simulink subsystem "rotorTemp"  (R2022b)
settings: Solver=VariableStepAuto  StartTime=0.0  StopTime=10.0  RelTol=1e-3
libraries: rotors x4
settings Model: Creator=serga  LastModifiedBy=serga

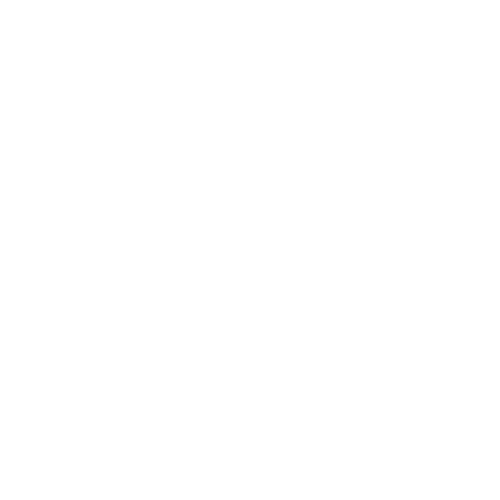
[thumbnail: Simulink's stored preview of the top-level diagram]
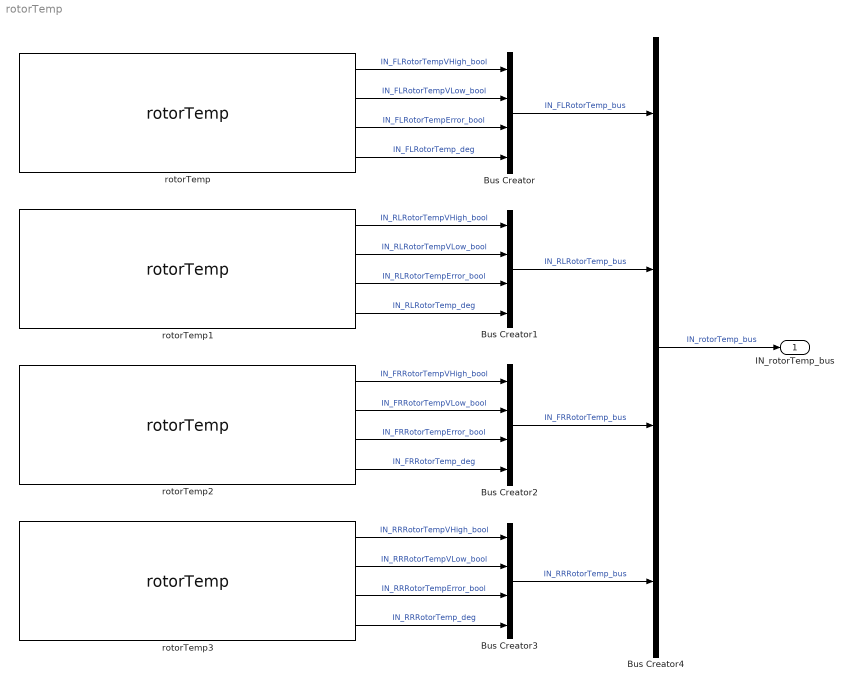
== system rotorTemp ==
  Bus Creator{,1..4} (5 alike) : BusCreator  Inputs=4
  rotorTemp : rotors/rotorTemp  pos='FL'
  rotorTemp1 : rotors/rotorTemp  pos='RL'
  rotorTemp2 : rotors/rotorTemp  pos='FR'
  rotorTemp3 : rotors/rotorTemp  pos='RR'
  IN_rotorTemp_bus : Outport
  wires:
  rotorTemp/1 -> Bus Creator/1  "IN_FLRotorTempVHigh_bool"
  rotorTemp/2 -> Bus Creator/2  "IN_FLRotorTempVLow_bool"
  rotorTemp/3 -> Bus Creator/3  "IN_FLRotorTempError_bool"
  rotorTemp/4 -> Bus Creator/4  "IN_FLRotorTemp_deg"
  rotorTemp1/1 -> Bus Creator1/1  "IN_RLRotorTempVHigh_bool"
  rotorTemp1/2 -> Bus Creator1/2  "IN_RLRotorTempVLow_bool"
  rotorTemp1/3 -> Bus Creator1/3  "IN_RLRotorTempError_bool"
  rotorTemp1/4 -> Bus Creator1/4  "IN_RLRotorTemp_deg"
  rotorTemp2/1 -> Bus Creator2/1  "IN_FRRotorTempVHigh_bool"
  rotorTemp2/2 -> Bus Creator2/2  "IN_FRRotorTempVLow_bool"
  rotorTemp2/3 -> Bus Creator2/3  "IN_FRRotorTempError_bool"
  rotorTemp2/4 -> Bus Creator2/4  "IN_FRRotorTemp_deg"
  rotorTemp3/1 -> Bus Creator3/1  "IN_RRRotorTempVHigh_bool"
  rotorTemp3/2 -> Bus Creator3/2  "IN_RRRotorTempVLow_bool"
  rotorTemp3/3 -> Bus Creator3/3  "IN_RRRotorTempError_bool"
  rotorTemp3/4 -> Bus Creator3/4  "IN_RRRotorTemp_deg"
  Bus Creator/1 -> Bus Creator4/1  "IN_FLRotorTemp_bus"
  Bus Creator1/1 -> Bus Creator4/2  "IN_RLRotorTemp_bus"
  Bus Creator2/1 -> Bus Creator4/3  "IN_FRRotorTemp_bus"
  Bus Creator3/1 -> Bus Creator4/4  "IN_RRRotorTemp_bus"
  Bus Creator4/1 -> IN_rotorTemp_bus/1  "IN_rotorTemp_bus"
